simulink model "Linear_MPC_design"  (R2021b)
settings: Solver=VariableStepAuto  StartTime=0.0  StopTime=10  RelTol=1e-3
libraries: cstblocks x1, mpclib x1
settings Model: Creator=PHAM DINH THANG  LastModifiedBy=PHAM DINH THANG

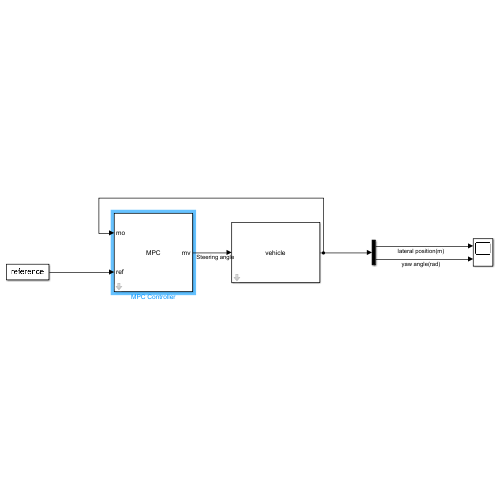
[thumbnail: Simulink's stored preview of the top-level diagram]
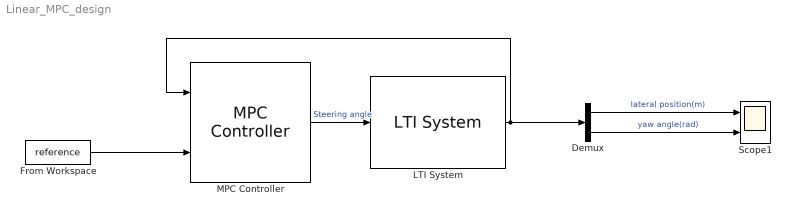
== system Linear_MPC_design ==
  Demux : Demux  Outputs=2
  From Workspace : FromWorkspace  VariableName=reference
  LTI System : cstblocks/LTI System  sys=vehicle  IC=[]
  MPC Controller : mpclib/MPC Controller  SCDEnableBlockLinearizationSpecification=on  is_multiple=0  enable_value=0  return_u0=off  updateMPCinCallerWorkspace=on  md_inport=off  mv_inport=off  uref_inport=off  return_cost=off  return_mvseq=off  return_qpstatus=off  return_xseq=off  return_state=off  return_ovseq=off  state_inport=off  umin_inport=off  umax_inport=off  ymin_inport=off  ymax_inport=off  cc_inport=off  ywt_inport=off  uwt_inport=off  duwt_inport=off  rhoeps_inport=off  pm_inport=off  MaximumP=10  HorizonChoice=FixedHorizon  n_ts=1  n_p=10  n_mv=1  n_md=1  n_ud=0  n_mo=2  n_uo=0  BlockDataType=double  SampleTimeInherited=off  switch_inport=off
  Scope1 : Scope  NumInputPorts=2
  wires:
  Demux/2 -> Scope1/2  "yaw angle(rad)"
  LTI System/1 -> MPC Controller/1, Demux/1
  Demux/1 -> Scope1/1  "lateral position(m)"
  From Workspace/1 -> MPC Controller/2
  MPC Controller/1 -> LTI System/1  "Steering angle"
